simulink model "SimulinkOminidirectinalDrone"  (R2025a)
settings: Solver=VariableStepAuto  StartTime=0.0  StopTime=10.0  RelTol=1e-3
values from neighbouring files (symbols this model uses):
  Cq = 0.0013    [TiltQua.m]
  Ct = 0.013    [TiltQua.m]
  g = 9.81    [TiltQua.m]
  H = 0.05    [B_matrix.m]
  Ixx = 0.1    [TiltQua.m]
  Iyy = 0.1    [TiltQua.m]
  Izz = 0.2    [TiltQua.m]
  L = 0.25    [B_matrix.m]
  rho = 1.225    [TiltQua.m]
undefined symbols (not defined in the file or in its folder): AUM, R_rad
libraries: sharedutil x4, aerolibobsolete x1
settings Model: Creator=Nguyen_Duc  LastModifiedBy=Admin
settings RTWCC: GPUComputeCapability=3.5

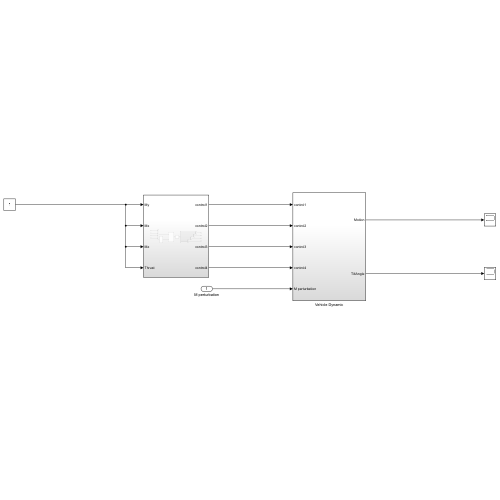
[thumbnail: Simulink's stored preview of the top-level diagram]
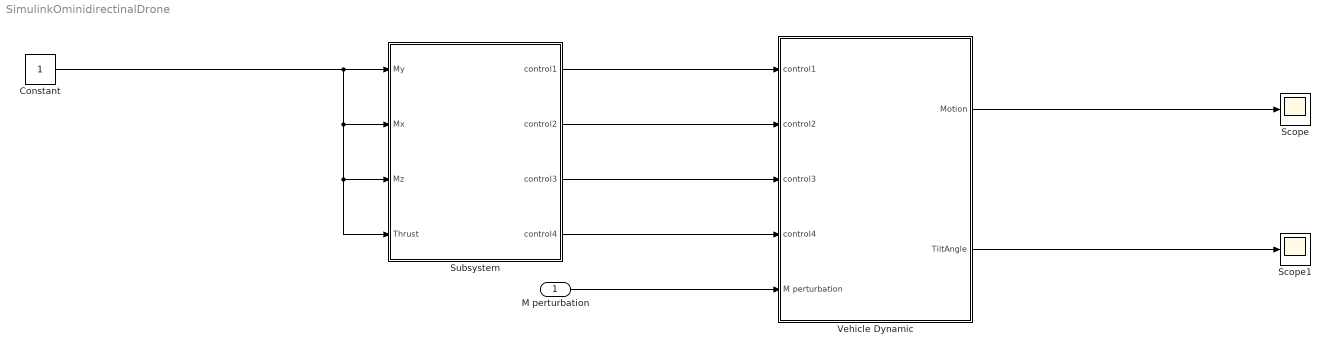
== system SimulinkOminidirectinalDrone ==
  M perturbation : Inport
  Constant : Constant
  Scope : Scope
  Scope1 : Scope
  Subsystem : Subsystem
  Vehicle Dynamic : Subsystem
  wires:
  Subsystem/1(control1) -> Vehicle Dynamic/1(control1)
  Subsystem/2(control2) -> Vehicle Dynamic/2(control2)
  Subsystem/3(control3) -> Vehicle Dynamic/3(control3)
  Subsystem/4(control4) -> Vehicle Dynamic/4(control4)
  M perturbation/1 -> Vehicle Dynamic/5(M perturbation)
  Vehicle Dynamic/1(Motion) -> Scope/1
  Vehicle Dynamic/2(TiltAngle) -> Scope1/1
  Constant/1 -> Subsystem/1(My), Subsystem/4(Thrust), Subsystem/3(Mz), Subsystem/2(Mx)

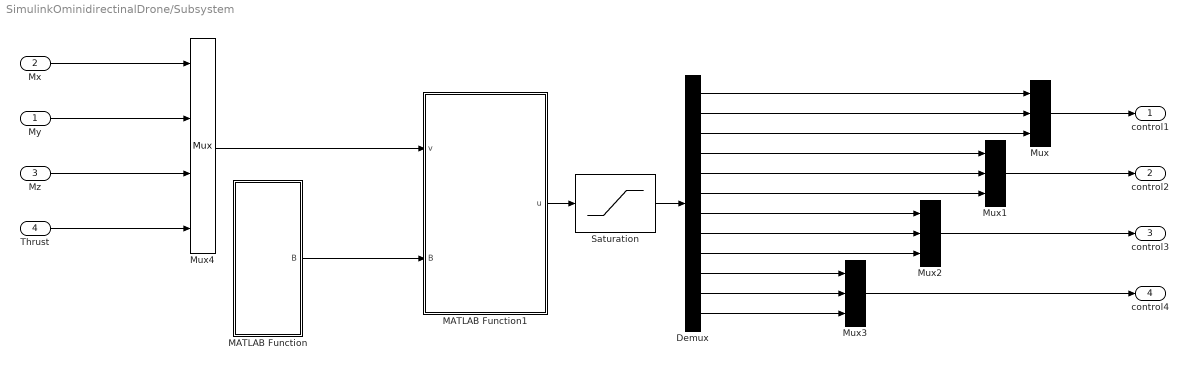
== system SimulinkOminidirectinalDrone/Subsystem ==
  My : Inport
  Mx : Inport  Port=2
  Mz : Inport  Port=3
  Thrust : Inport  Port=4
  Demux : Demux  Outputs=12
  MATLAB Function : MATLAB Function  TreatAsAtomicUnit=on
  MATLAB Function1 : MATLAB Function  TreatAsAtomicUnit=on
  Mux{,1..3} (4 alike) : Mux  Inputs=3
  Mux4 : Mux
  Saturation : Saturate  UpperLimit="[1  30*pi/180  0.2  1  30*pi/180  0.2  1  30*pi/180  0.2  1  30*pi/180  0.2]"  LowerLimit="[0 -30*pi/180 -0.2  0 -30*pi/180 -0.2  0 -30*pi/180 -0.2  0 -30*pi/180 -0.2]"
  control1 : Outport
  control2 : Outport  Port=2
  control3 : Outport  Port=3
  control4 : Outport  Port=4
  wires:
  MATLAB Function/1(B) -> MATLAB Function1/2(B)
  Mux4/1 -> MATLAB Function1/1(v)
  MATLAB Function1/1(u) -> Saturation/1
  Saturation/1 -> Demux/1
  Demux/1 -> Mux/1
  Mux/1 -> control1/1
  Demux/3 -> Mux/3
  Demux/2 -> Mux/2
  Demux/4 -> Mux1/1
  Demux/5 -> Mux1/2
  Demux/6 -> Mux1/3
  Demux/7 -> Mux2/1
  Demux/8 -> Mux2/2
  Demux/9 -> Mux2/3
  Demux/10 -> Mux3/1
  Demux/11 -> Mux3/2
  Demux/12 -> Mux3/3
  Mux1/1 -> control2/1
  Mux2/1 -> control3/1
  Mux3/1 -> control4/1
  Mx/1 -> Mux4/1
  My/1 -> Mux4/2
  Mz/1 -> Mux4/3
  Thrust/1 -> Mux4/4

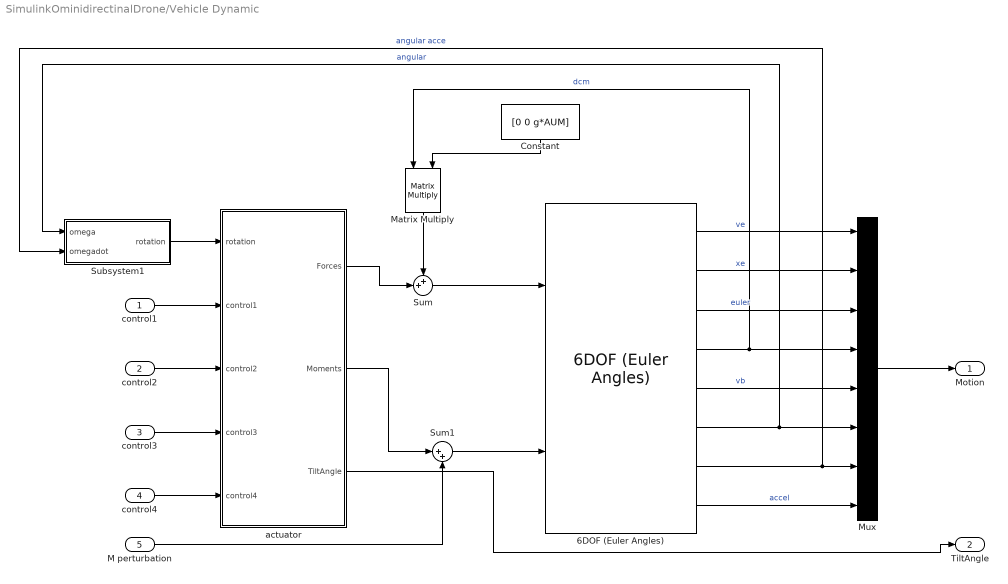
== system SimulinkOminidirectinalDrone/Vehicle Dynamic ==
  control1 : Inport
  control2 : Inport  Port=2
  control3 : Inport  Port=3
  control4 : Inport  Port=4
  M perturbation : Inport  Port=5
  6DOF (Euler Angles) : aerolibobsolete/6DOF (Euler Angles)  units=Metric (MKS)  mtype=Fixed  rep=Euler Angles  xme_0=[0 0 0]  Vm_0=[0 0 0]  eul_0=[0 0 0]  pm_0=[0 0 0]  mass_0=1.0  mass_e=0.5  mass_f=2.0  inertia=eye(3)  inertia_e=eye(3)  inertia_f=2*eye(3)  k_quat=1.0  vre_flag=on  abi_flag=off  aMode=0  xme_statename=''  Vm_statename=''  eul_statename=''  quat_statename=''  pm_statename=''  mass_statename=''
  Constant : Constant  Value=[0 0 g*AUM]
  Matrix Multiply : Product  Multiplication=Matrix(*)
  Mux : Mux  Inputs=8
  Subsystem1 : Subsystem
  Sum : Sum  Inputs=++|
  Sum1 : Sum  Inputs=|++
  actuator : Subsystem
  Motion : Outport
  TiltAngle : Outport  Port=2
  wires:
  control3/1 -> actuator/4(control3)
  M perturbation/1 -> Sum1/2
  Matrix Multiply/1 -> Sum/1
  6DOF (Euler Angles)/7 -> Subsystem1/2(omegadot), Mux/7  "angular acce"
  6DOF (Euler Angles)/3 -> Mux/3  "euler"
  Mux/1 -> Motion/1
  control1/1 -> actuator/2(control1)
  6DOF (Euler Angles)/2 -> Mux/2  "xe"
  6DOF (Euler Angles)/1 -> Mux/1  "ve"
  control2/1 -> actuator/3(control2)
  control4/1 -> actuator/5(control4)
  Constant/1 -> Matrix Multiply/2
  6DOF (Euler Angles)/8 -> Mux/8  "accel"
  6DOF (Euler Angles)/6 -> Subsystem1/1(omega), Mux/6  "angular"
  6DOF (Euler Angles)/5 -> Mux/5  "vb"
  6DOF (Euler Angles)/4 -> Matrix Multiply/1, Mux/4  "dcm"
  Sum1/1 -> 6DOF (Euler Angles)/2
  actuator/3(TiltAngle) -> TiltAngle/1
  Subsystem1/1(rotation) -> actuator/1(rotation)
  Sum/1 -> 6DOF (Euler Angles)/1
  actuator/1(Forces) -> Sum/2
  actuator/2(Moments) -> Sum1/1

== system SimulinkOminidirectinalDrone/Vehicle Dynamic/Subsystem1 ==
  omega : Inport
  omegadot : Inport  Port=2
  Demux : Demux  Outputs=3
  Demux1 : Demux  Outputs=3
  Mux1 : Mux  Inputs=6
  rotation : Outport
  wires:
  Mux1/1 -> rotation/1
  Demux/3 -> Mux1/3
  Demux1/1 -> Mux1/4
  omega/1 -> Demux/1
  Demux1/2 -> Mux1/5
  Demux/1 -> Mux1/1
  Demux/2 -> Mux1/2
  omegadot/1 -> Demux1/1
  Demux1/3 -> Mux1/6

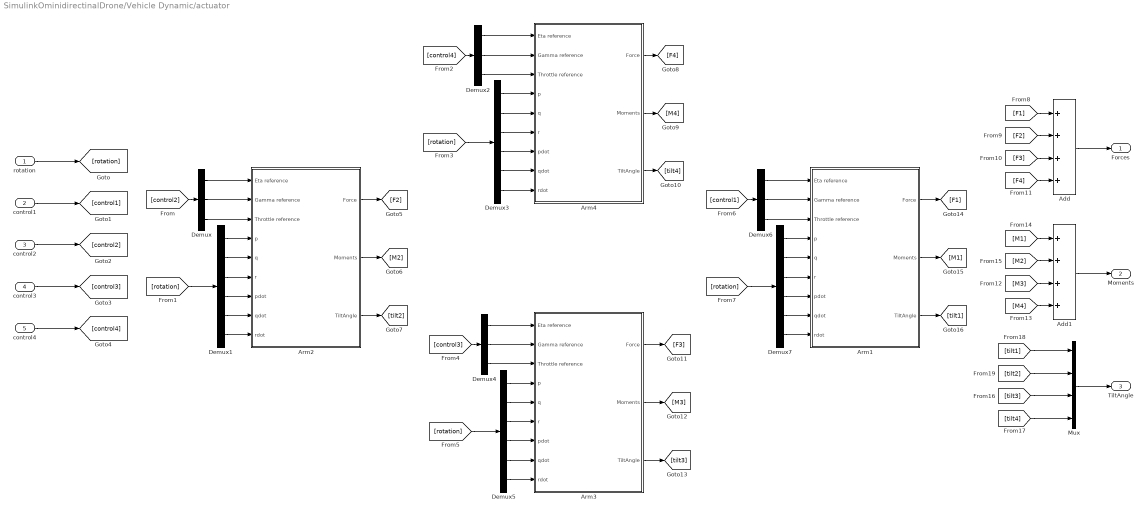
== system SimulinkOminidirectinalDrone/Vehicle Dynamic/actuator ==
  rotation : Inport
  control1 : Inport  Port=2
  control2 : Inport  Port=3
  control3 : Inport  Port=4
  control4 : Inport  Port=5
  Add : Sum  Inputs=++++
  Add1 : Sum  Inputs=++++
  Arm1 : Subsystem
  Arm2 : Subsystem
  Arm3 : Subsystem
  Arm4 : Subsystem
  Demux{,2,4,6} (4 alike) : Demux  Outputs=3
  Demux{1,3,5,7} (4 alike) : Demux  Outputs=6
  Mux : Mux
  Forces : Outport
  Moments : Outport  Port=2
  TiltAngle : Outport  Port=3
  wires:
  Demux5/3 -> Arm3/6(r)
  Demux7/6 -> Arm1/9(rdot)
  control3/1 -> [control3]
  Demux1/3 -> Arm2/6(r)
  Demux6/2 -> Arm1/2(Gamma reference)
  Add/1 -> Forces/1
  Demux4/3 -> Arm3/3(Throttle reference)
  Demux2/3 -> Arm4/3(Throttle reference)
  [F4] -> Add/4
  Arm1/3(TiltAngle) -> [tilt1]
  [tilt4] -> Mux/4
  [M3] -> Add1/3
  Demux4/2 -> Arm3/2(Gamma reference)
  Demux5/2 -> Arm3/5(q)
  [control1] -> Demux6/1
  Arm1/2(Moments) -> [M1]
  Arm3/1(Force) -> [F3]
  Demux7/3 -> Arm1/6(r)
  Demux5/5 -> Arm3/8(qdot)
  [M2] -> Add1/2
  Arm2/1(Force) -> [F2]
  Arm1/1(Force) -> [F1]
  Demux1/2 -> Arm2/5(q)
  Demux7/5 -> Arm1/8(qdot)
  Demux1/6 -> Arm2/9(rdot)
  [rotation] -> Demux3/1
  [M1] -> Add1/1
  [M4] -> Add1/4
  [control3] -> Demux4/1
  Add1/1 -> Moments/1
  Demux5/6 -> Arm3/9(rdot)
  Demux3/2 -> Arm4/5(q)
  [tilt2] -> Mux/2
  Demux1/1 -> Arm2/4(p)
  Arm4/1(Force) -> [F4]
  Demux5/4 -> Arm3/7(pdot)
  Demux3/5 -> Arm4/8(qdot)
  Demux3/4 -> Arm4/7(pdot)
  Demux3/6 -> Arm4/9(rdot)
  Demux6/1 -> Arm1/1(Eta reference)
  Demux7/2 -> Arm1/5(q)
  Arm3/2(Moments) -> [M3]
  Demux7/4 -> Arm1/7(pdot)
  Arm4/2(Moments) -> [M4]
  control1/1 -> [control1]
  Demux2/2 -> Arm4/2(Gamma reference)
  Arm2/3(TiltAngle) -> [tilt2]
  [control4] -> Demux2/1
  Demux3/3 -> Arm4/6(r)
  Demux3/1 -> Arm4/4(p)
  Demux6/3 -> Arm1/3(Throttle reference)
  Arm4/3(TiltAngle) -> [tilt4]
  Demux2/1 -> Arm4/1(Eta reference)
  Demux5/1 -> Arm3/4(p)
  Demux/2 -> Arm2/2(Gamma reference)
  [control2] -> Demux/1
  control2/1 -> [control2]
  Demux7/1 -> Arm1/4(p)
  Arm2/2(Moments) -> [M2]
  [rotation] -> Demux1/1
  Arm3/3(TiltAngle) -> [tilt3]
  [rotation] -> Demux7/1
  Demux/1 -> Arm2/1(Eta reference)
  Demux4/1 -> Arm3/1(Eta reference)
  [rotation] -> Demux5/1
  Demux1/4 -> Arm2/7(pdot)
  rotation/1 -> [rotation]
  Demux/3 -> Arm2/3(Throttle reference)
  control4/1 -> [control4]
  Demux1/5 -> Arm2/8(qdot)
  Mux/1 -> TiltAngle/1
  [F3] -> Add/3
  [F1] -> Add/1
  [tilt1] -> Mux/1
  [tilt3] -> Mux/3
  [F2] -> Add/2

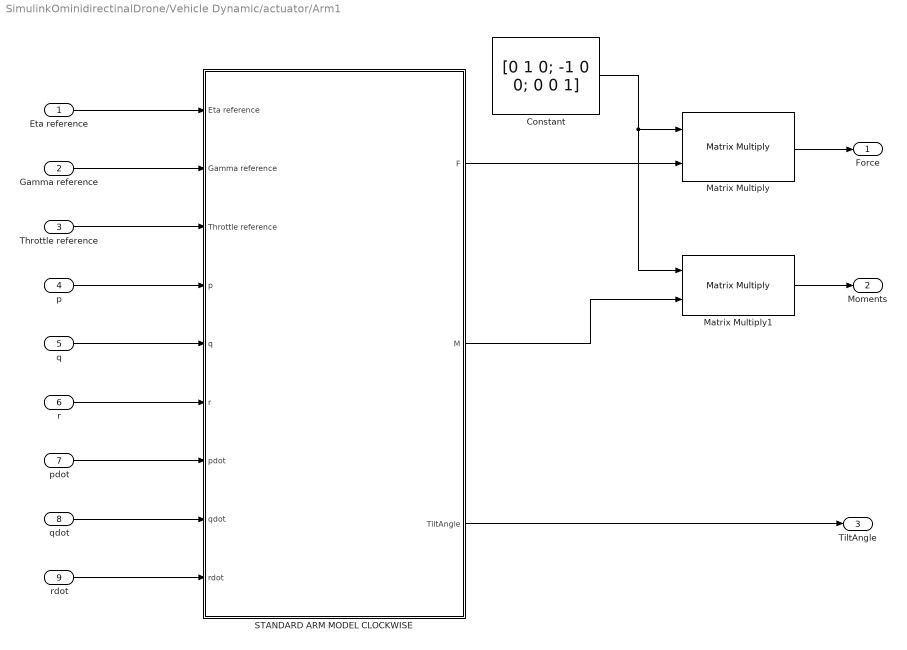
== system SimulinkOminidirectinalDrone/Vehicle Dynamic/actuator/Arm1 ==
  Eta reference : Inport
  Gamma reference : Inport  Port=2
  Throttle reference : Inport  Port=3
  p : Inport  Port=4
  q : Inport  Port=5
  r : Inport  Port=6
  pdot : Inport  Port=7
  qdot : Inport  Port=8
  rdot : Inport  Port=9
  Constant : Constant  Value=[0 1 0; -1 0 0; 0 0 1]
  Matrix Multiply : Product  Multiplication=Matrix(*)
  Matrix Multiply1 : Product  Multiplication=Matrix(*)
  STANDARD ARM MODEL CLOCKWISE : Subsystem
  Force : Outport
  Moments : Outport  Port=2
  TiltAngle : Outport  Port=3
  wires:
  Gamma reference/1 -> STANDARD ARM MODEL CLOCKWISE/2(Gamma reference)
  Eta reference/1 -> STANDARD ARM MODEL CLOCKWISE/1(Eta reference)
  Matrix Multiply1/1 -> Moments/1
  STANDARD ARM MODEL CLOCKWISE/1(F) -> Matrix Multiply/2
  Throttle reference/1 -> STANDARD ARM MODEL CLOCKWISE/3(Throttle reference)
  r/1 -> STANDARD ARM MODEL CLOCKWISE/6(r)
  p/1 -> STANDARD ARM MODEL CLOCKWISE/4(p)
  q/1 -> STANDARD ARM MODEL CLOCKWISE/5(q)
  STANDARD ARM MODEL CLOCKWISE/2(M) -> Matrix Multiply1/2
  pdot/1 -> STANDARD ARM MODEL CLOCKWISE/7(pdot)
  qdot/1 -> STANDARD ARM MODEL CLOCKWISE/8(qdot)
  rdot/1 -> STANDARD ARM MODEL CLOCKWISE/9(rdot)
  Constant/1 -> Matrix Multiply1/1, Matrix Multiply/1
  Matrix Multiply/1 -> Force/1
  STANDARD ARM MODEL CLOCKWISE/3(TiltAngle) -> TiltAngle/1

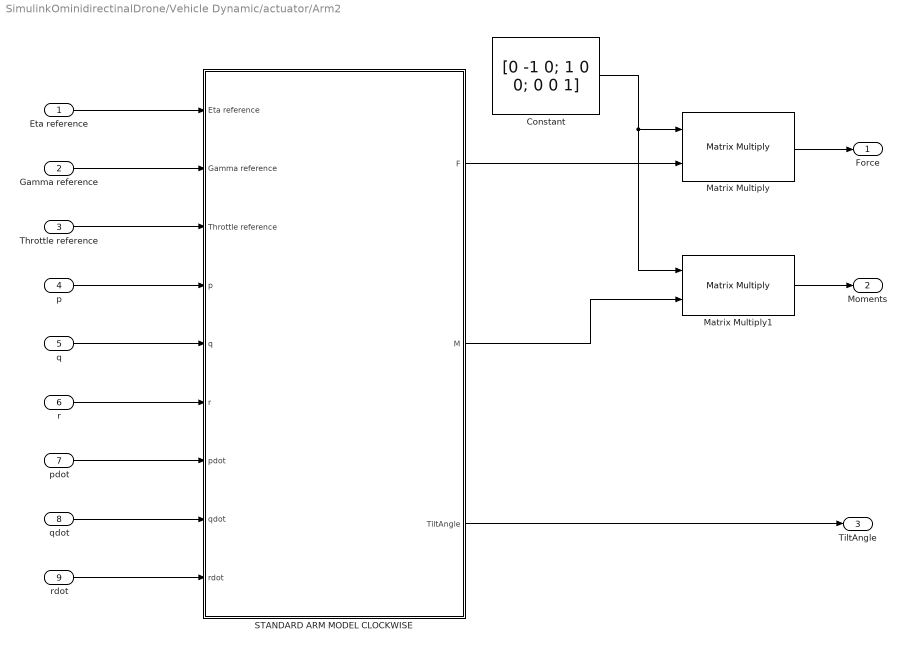
== system SimulinkOminidirectinalDrone/Vehicle Dynamic/actuator/Arm2 ==
  Eta reference : Inport
  Gamma reference : Inport  Port=2
  Throttle reference : Inport  Port=3
  p : Inport  Port=4
  q : Inport  Port=5
  r : Inport  Port=6
  pdot : Inport  Port=7
  qdot : Inport  Port=8
  rdot : Inport  Port=9
  Constant : Constant  Value=[0 -1 0; 1 0 0; 0 0 1]
  Matrix Multiply : Product  Multiplication=Matrix(*)
  Matrix Multiply1 : Product  Multiplication=Matrix(*)
  STANDARD ARM MODEL CLOCKWISE : Subsystem
  Force : Outport
  Moments : Outport  Port=2
  TiltAngle : Outport  Port=3
  wires:
  Gamma reference/1 -> STANDARD ARM MODEL CLOCKWISE/2(Gamma reference)
  Eta reference/1 -> STANDARD ARM MODEL CLOCKWISE/1(Eta reference)
  Matrix Multiply1/1 -> Moments/1
  STANDARD ARM MODEL CLOCKWISE/1(F) -> Matrix Multiply/2
  Throttle reference/1 -> STANDARD ARM MODEL CLOCKWISE/3(Throttle reference)
  r/1 -> STANDARD ARM MODEL CLOCKWISE/6(r)
  p/1 -> STANDARD ARM MODEL CLOCKWISE/4(p)
  q/1 -> STANDARD ARM MODEL CLOCKWISE/5(q)
  STANDARD ARM MODEL CLOCKWISE/2(M) -> Matrix Multiply1/2
  pdot/1 -> STANDARD ARM MODEL CLOCKWISE/7(pdot)
  qdot/1 -> STANDARD ARM MODEL CLOCKWISE/8(qdot)
  rdot/1 -> STANDARD ARM MODEL CLOCKWISE/9(rdot)
  Constant/1 -> Matrix Multiply1/1, Matrix Multiply/1
  Matrix Multiply/1 -> Force/1
  STANDARD ARM MODEL CLOCKWISE/3(TiltAngle) -> TiltAngle/1

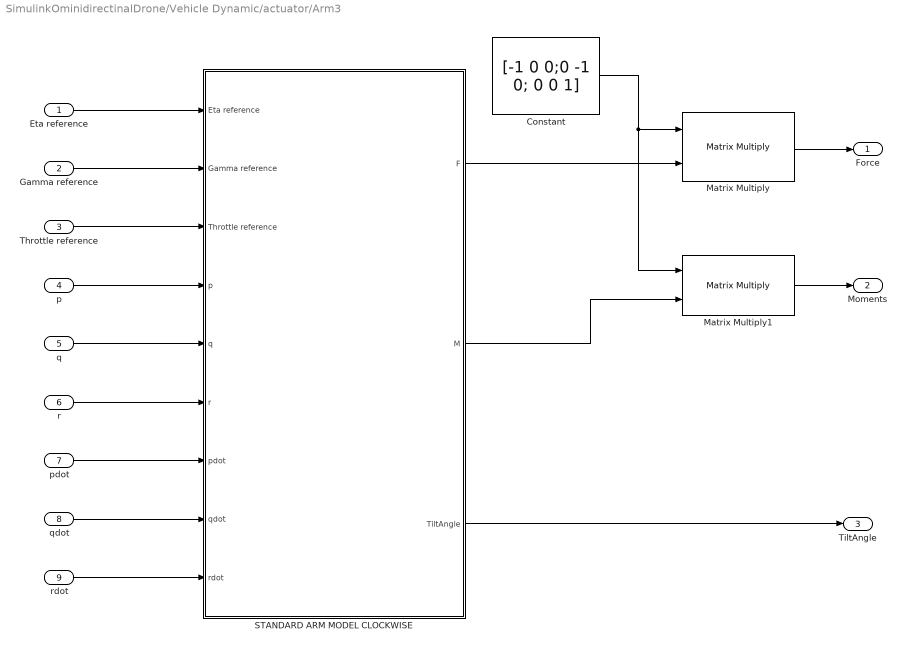
== system SimulinkOminidirectinalDrone/Vehicle Dynamic/actuator/Arm3 ==
  Eta reference : Inport
  Gamma reference : Inport  Port=2
  Throttle reference : Inport  Port=3
  p : Inport  Port=4
  q : Inport  Port=5
  r : Inport  Port=6
  pdot : Inport  Port=7
  qdot : Inport  Port=8
  rdot : Inport  Port=9
  Constant : Constant  Value=[-1 0 0;0 -1 0; 0 0 1]
  Matrix Multiply : Product  Multiplication=Matrix(*)
  Matrix Multiply1 : Product  Multiplication=Matrix(*)
  STANDARD ARM MODEL CLOCKWISE : Subsystem
  Force : Outport
  Moments : Outport  Port=2
  TiltAngle : Outport  Port=3
  wires:
  Gamma reference/1 -> STANDARD ARM MODEL CLOCKWISE/2(Gamma reference)
  Eta reference/1 -> STANDARD ARM MODEL CLOCKWISE/1(Eta reference)
  Matrix Multiply1/1 -> Moments/1
  STANDARD ARM MODEL CLOCKWISE/1(F) -> Matrix Multiply/2
  Throttle reference/1 -> STANDARD ARM MODEL CLOCKWISE/3(Throttle reference)
  r/1 -> STANDARD ARM MODEL CLOCKWISE/6(r)
  p/1 -> STANDARD ARM MODEL CLOCKWISE/4(p)
  q/1 -> STANDARD ARM MODEL CLOCKWISE/5(q)
  STANDARD ARM MODEL CLOCKWISE/2(M) -> Matrix Multiply1/2
  pdot/1 -> STANDARD ARM MODEL CLOCKWISE/7(pdot)
  qdot/1 -> STANDARD ARM MODEL CLOCKWISE/8(qdot)
  rdot/1 -> STANDARD ARM MODEL CLOCKWISE/9(rdot)
  Constant/1 -> Matrix Multiply1/1, Matrix Multiply/1
  Matrix Multiply/1 -> Force/1
  STANDARD ARM MODEL CLOCKWISE/3(TiltAngle) -> TiltAngle/1

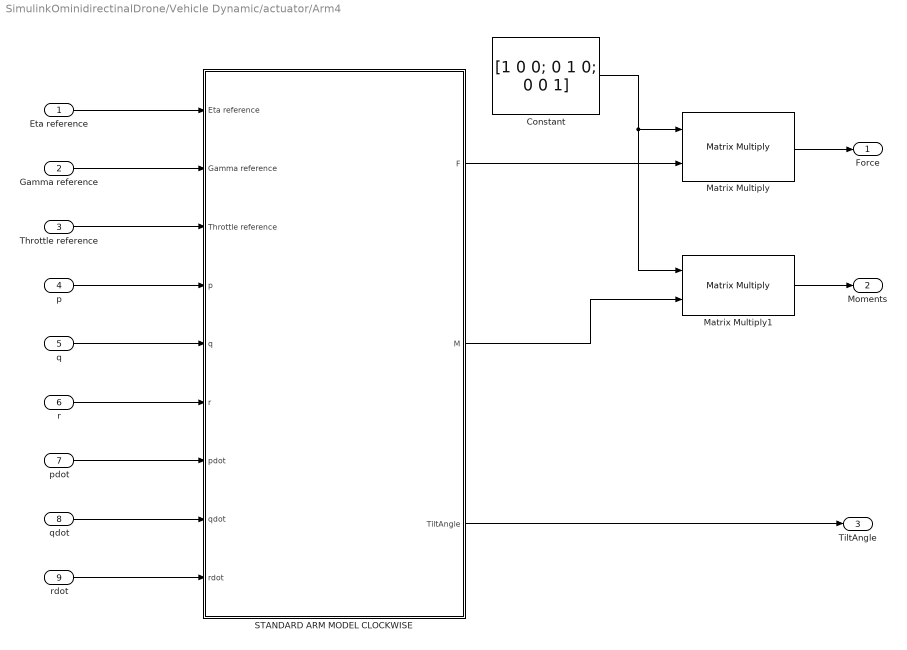
== system SimulinkOminidirectinalDrone/Vehicle Dynamic/actuator/Arm4 ==
  Eta reference : Inport
  Gamma reference : Inport  Port=2
  Throttle reference : Inport  Port=3
  p : Inport  Port=4
  q : Inport  Port=5
  r : Inport  Port=6
  pdot : Inport  Port=7
  qdot : Inport  Port=8
  rdot : Inport  Port=9
  Constant : Constant  Value=[1 0 0; 0 1 0; 0 0 1]
  Matrix Multiply : Product  Multiplication=Matrix(*)
  Matrix Multiply1 : Product  Multiplication=Matrix(*)
  STANDARD ARM MODEL CLOCKWISE : Subsystem
  Force : Outport
  Moments : Outport  Port=2
  TiltAngle : Outport  Port=3
  wires:
  Gamma reference/1 -> STANDARD ARM MODEL CLOCKWISE/2(Gamma reference)
  Eta reference/1 -> STANDARD ARM MODEL CLOCKWISE/1(Eta reference)
  Matrix Multiply1/1 -> Moments/1
  STANDARD ARM MODEL CLOCKWISE/1(F) -> Matrix Multiply/2
  Throttle reference/1 -> STANDARD ARM MODEL CLOCKWISE/3(Throttle reference)
  r/1 -> STANDARD ARM MODEL CLOCKWISE/6(r)
  p/1 -> STANDARD ARM MODEL CLOCKWISE/4(p)
  q/1 -> STANDARD ARM MODEL CLOCKWISE/5(q)
  STANDARD ARM MODEL CLOCKWISE/2(M) -> Matrix Multiply1/2
  pdot/1 -> STANDARD ARM MODEL CLOCKWISE/7(pdot)
  qdot/1 -> STANDARD ARM MODEL CLOCKWISE/8(qdot)
  rdot/1 -> STANDARD ARM MODEL CLOCKWISE/9(rdot)
  Constant/1 -> Matrix Multiply1/1, Matrix Multiply/1
  Matrix Multiply/1 -> Force/1
  STANDARD ARM MODEL CLOCKWISE/3(TiltAngle) -> TiltAngle/1

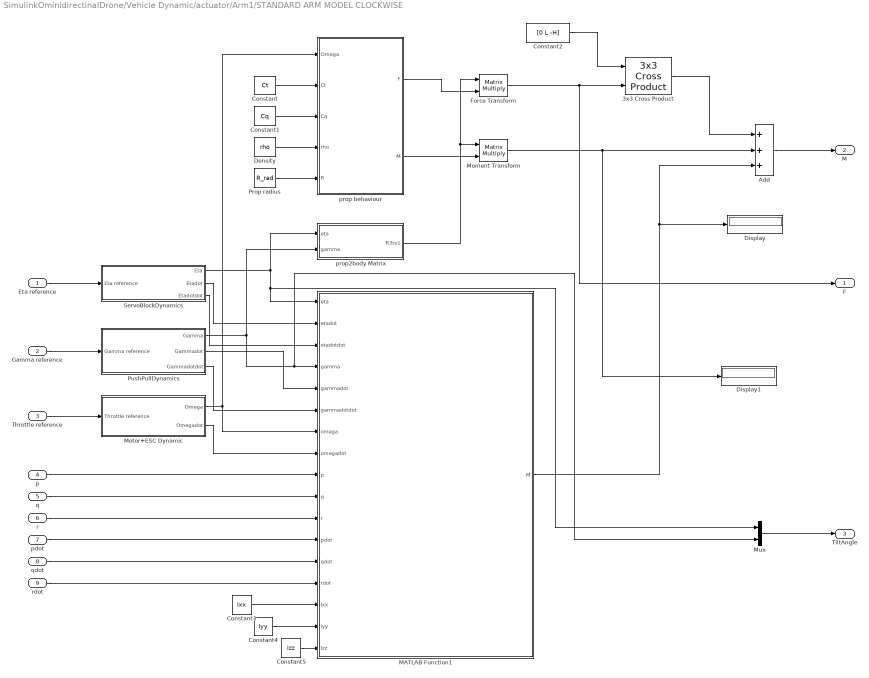
== system SimulinkOminidirectinalDrone/Vehicle Dynamic/actuator/Arm1/STANDARD ARM MODEL CLOCKWISE ==
  Eta reference : Inport
  Gamma reference : Inport  Port=2
  Throttle reference : Inport  Port=3
  p : Inport  Port=4
  q : Inport  Port=5
  r : Inport  Port=6
  pdot : Inport  Port=7
  qdot : Inport  Port=8
  rdot : Inport  Port=9
  3x3 Cross Product : sharedutil/3x3 Cross Product  aMode=aMode
      settings: LibrarySourceBlock=aerolibutil/3x3 Cross Product
  Add : Sum  Inputs=+++
  Constant : Constant  Value=Ct
  Constant1 : Constant  Value=Cq
  Constant2 : Constant  Value=[0 L -H]
  Constant3 : Constant  Value=Ixx
  Constant4 : Constant  Value=Iyy
  Constant5 : Constant  Value=Izz
  Density : Constant  Value=rho
  Display : Display
  Display1 : Display
  Force Transform : Product  Multiplication=Matrix(*)
  MATLAB Function1 : MATLAB Function  TreatAsAtomicUnit=on
  Moment Transform : Product  Multiplication=Matrix(*)
  Motor+ESC Dynamic : Subsystem
  Mux : Mux  Inputs=2
  Prop radius : Constant  Value=R_rad
  PushPullDynamics : Subsystem
  ServoBlockDynamics : Subsystem
  prop behaviour : MATLAB Function  TreatAsAtomicUnit=on
  prop2body Matrix : MATLAB Function  TreatAsAtomicUnit=on
  F : Outport
  M : Outport  Port=2
  TiltAngle : Outport  Port=3
  wires:
  Motor+ESC Dynamic/2(Omegadot) -> MATLAB Function1/8(omegadot)
  PushPullDynamics/3(Gammadotdot) -> MATLAB Function1/6(gammadotdot)
  Constant5/1 -> MATLAB Function1/17(Izz)
  Constant4/1 -> MATLAB Function1/16(Iyy)
  p/1 -> MATLAB Function1/9(p)
  prop2body Matrix/1(R3to1) -> Moment Transform/1, Force Transform/1
  Moment Transform/1 -> Display1/1, Add/2
  Prop radius/1 -> prop behaviour/5(R)
  Gamma reference/1 -> PushPullDynamics/1(Gamma reference)
  qdot/1 -> MATLAB Function1/13(qdot)
  Constant1/1 -> prop behaviour/3(Cq)
  Throttle reference/1 -> Motor+ESC Dynamic/1(Throttle reference)
  3x3 Cross Product/1 -> Add/1
  q/1 -> MATLAB Function1/10(q)
  Density/1 -> prop behaviour/4(rho)
  Motor+ESC Dynamic/1(Omega) -> MATLAB Function1/7(omega), prop behaviour/1(Omega)
  ServoBlockDynamics/3(Etadotdot) -> MATLAB Function1/3(etadotdot)
  prop behaviour/2(M) -> Moment Transform/2
  Constant3/1 -> MATLAB Function1/15(Ixx)
  PushPullDynamics/1(Gamma) -> Mux/2, MATLAB Function1/4(gamma), prop2body Matrix/2(gamma)
  Constant2/1 -> 3x3 Cross Product/1
  Force Transform/1 -> F/1, 3x3 Cross Product/2
  MATLAB Function1/1(M) -> Display/1, Add/3
  ServoBlockDynamics/1(Eta) -> Mux/1, MATLAB Function1/1(eta), prop2body Matrix/1(eta)
  r/1 -> MATLAB Function1/11(r)
  rdot/1 -> MATLAB Function1/14(rdot)
  Eta reference/1 -> ServoBlockDynamics/1(Eta reference)
  Mux/1 -> TiltAngle/1
  PushPullDynamics/2(Gammadot) -> MATLAB Function1/5(gammadot)
  pdot/1 -> MATLAB Function1/12(pdot)
  prop behaviour/1(F) -> Force Transform/2
  Constant/1 -> prop behaviour/2(Ct)
  Add/1 -> M/1
  ServoBlockDynamics/2(Etadot) -> MATLAB Function1/2(etadot)

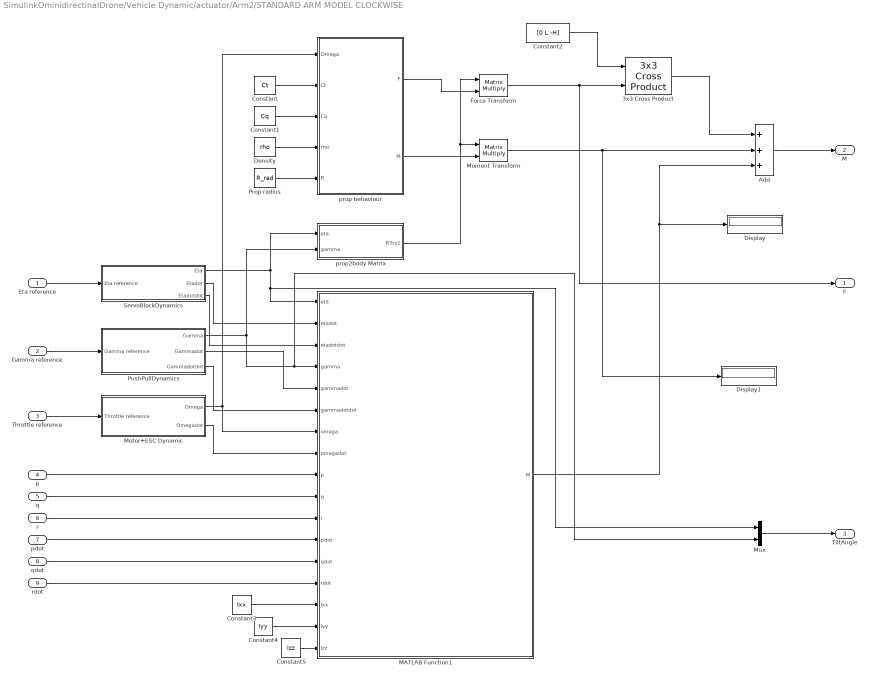
== system SimulinkOminidirectinalDrone/Vehicle Dynamic/actuator/Arm2/STANDARD ARM MODEL CLOCKWISE ==
  Eta reference : Inport
  Gamma reference : Inport  Port=2
  Throttle reference : Inport  Port=3
  p : Inport  Port=4
  q : Inport  Port=5
  r : Inport  Port=6
  pdot : Inport  Port=7
  qdot : Inport  Port=8
  rdot : Inport  Port=9
  3x3 Cross Product : sharedutil/3x3 Cross Product  aMode=aMode
      settings: LibrarySourceBlock=aerolibutil/3x3 Cross Product
  Add : Sum  Inputs=+++
  Constant : Constant  Value=Ct
  Constant1 : Constant  Value=Cq
  Constant2 : Constant  Value=[0 L -H]
  Constant3 : Constant  Value=Ixx
  Constant4 : Constant  Value=Iyy
  Constant5 : Constant  Value=Izz
  Density : Constant  Value=rho
  Display : Display
  Display1 : Display
  Force Transform : Product  Multiplication=Matrix(*)
  MATLAB Function1 : MATLAB Function  TreatAsAtomicUnit=on
  Moment Transform : Product  Multiplication=Matrix(*)
  Motor+ESC Dynamic : Subsystem
  Mux : Mux  Inputs=2
  Prop radius : Constant  Value=R_rad
  PushPullDynamics : Subsystem
  ServoBlockDynamics : Subsystem
  prop behaviour : MATLAB Function  TreatAsAtomicUnit=on
  prop2body Matrix : MATLAB Function  TreatAsAtomicUnit=on
  F : Outport
  M : Outport  Port=2
  TiltAngle : Outport  Port=3
  wires:
  Motor+ESC Dynamic/2(Omegadot) -> MATLAB Function1/8(omegadot)
  PushPullDynamics/3(Gammadotdot) -> MATLAB Function1/6(gammadotdot)
  Constant5/1 -> MATLAB Function1/17(Izz)
  Constant4/1 -> MATLAB Function1/16(Iyy)
  p/1 -> MATLAB Function1/9(p)
  prop2body Matrix/1(R3to1) -> Moment Transform/1, Force Transform/1
  Moment Transform/1 -> Display1/1, Add/2
  Prop radius/1 -> prop behaviour/5(R)
  Gamma reference/1 -> PushPullDynamics/1(Gamma reference)
  qdot/1 -> MATLAB Function1/13(qdot)
  Constant1/1 -> prop behaviour/3(Cq)
  Throttle reference/1 -> Motor+ESC Dynamic/1(Throttle reference)
  3x3 Cross Product/1 -> Add/1
  q/1 -> MATLAB Function1/10(q)
  Density/1 -> prop behaviour/4(rho)
  Motor+ESC Dynamic/1(Omega) -> MATLAB Function1/7(omega), prop behaviour/1(Omega)
  ServoBlockDynamics/3(Etadotdot) -> MATLAB Function1/3(etadotdot)
  prop behaviour/2(M) -> Moment Transform/2
  Constant3/1 -> MATLAB Function1/15(Ixx)
  PushPullDynamics/1(Gamma) -> Mux/2, MATLAB Function1/4(gamma), prop2body Matrix/2(gamma)
  Constant2/1 -> 3x3 Cross Product/1
  Force Transform/1 -> F/1, 3x3 Cross Product/2
  MATLAB Function1/1(M) -> Display/1, Add/3
  ServoBlockDynamics/1(Eta) -> Mux/1, MATLAB Function1/1(eta), prop2body Matrix/1(eta)
  r/1 -> MATLAB Function1/11(r)
  rdot/1 -> MATLAB Function1/14(rdot)
  Eta reference/1 -> ServoBlockDynamics/1(Eta reference)
  Mux/1 -> TiltAngle/1
  PushPullDynamics/2(Gammadot) -> MATLAB Function1/5(gammadot)
  pdot/1 -> MATLAB Function1/12(pdot)
  prop behaviour/1(F) -> Force Transform/2
  Constant/1 -> prop behaviour/2(Ct)
  Add/1 -> M/1
  ServoBlockDynamics/2(Etadot) -> MATLAB Function1/2(etadot)

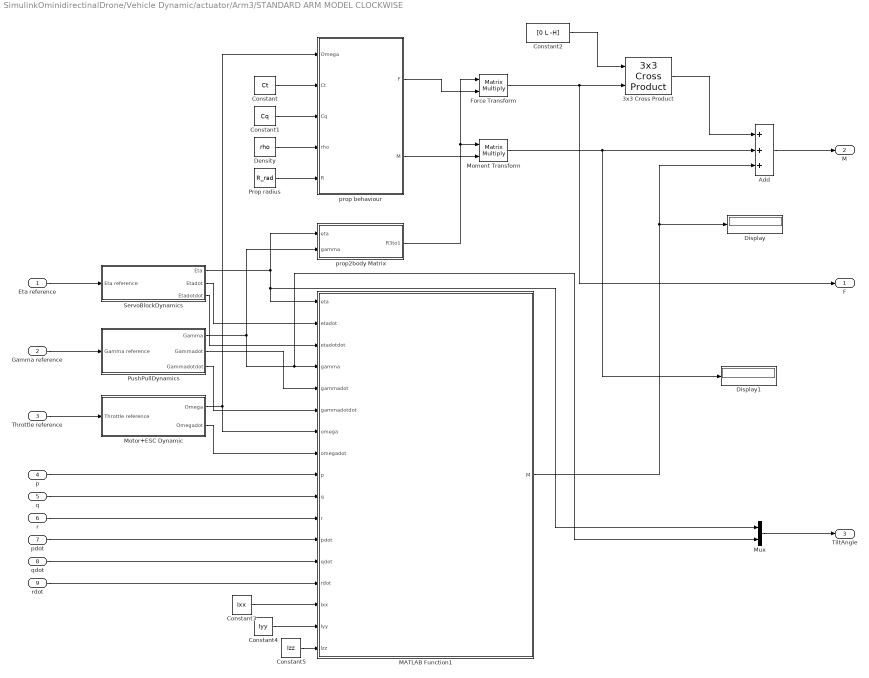
== system SimulinkOminidirectinalDrone/Vehicle Dynamic/actuator/Arm3/STANDARD ARM MODEL CLOCKWISE ==
  Eta reference : Inport
  Gamma reference : Inport  Port=2
  Throttle reference : Inport  Port=3
  p : Inport  Port=4
  q : Inport  Port=5
  r : Inport  Port=6
  pdot : Inport  Port=7
  qdot : Inport  Port=8
  rdot : Inport  Port=9
  3x3 Cross Product : sharedutil/3x3 Cross Product  aMode=aMode
      settings: LibrarySourceBlock=aerolibutil/3x3 Cross Product
  Add : Sum  Inputs=+++
  Constant : Constant  Value=Ct
  Constant1 : Constant  Value=Cq
  Constant2 : Constant  Value=[0 L -H]
  Constant3 : Constant  Value=Ixx
  Constant4 : Constant  Value=Iyy
  Constant5 : Constant  Value=Izz
  Density : Constant  Value=rho
  Display : Display
  Display1 : Display
  Force Transform : Product  Multiplication=Matrix(*)
  MATLAB Function1 : MATLAB Function  TreatAsAtomicUnit=on
  Moment Transform : Product  Multiplication=Matrix(*)
  Motor+ESC Dynamic : Subsystem
  Mux : Mux  Inputs=2
  Prop radius : Constant  Value=R_rad
  PushPullDynamics : Subsystem
  ServoBlockDynamics : Subsystem
  prop behaviour : MATLAB Function  TreatAsAtomicUnit=on
  prop2body Matrix : MATLAB Function  TreatAsAtomicUnit=on
  F : Outport
  M : Outport  Port=2
  TiltAngle : Outport  Port=3
  wires:
  Motor+ESC Dynamic/2(Omegadot) -> MATLAB Function1/8(omegadot)
  PushPullDynamics/3(Gammadotdot) -> MATLAB Function1/6(gammadotdot)
  Constant5/1 -> MATLAB Function1/17(Izz)
  Constant4/1 -> MATLAB Function1/16(Iyy)
  p/1 -> MATLAB Function1/9(p)
  prop2body Matrix/1(R3to1) -> Moment Transform/1, Force Transform/1
  Moment Transform/1 -> Display1/1, Add/2
  Prop radius/1 -> prop behaviour/5(R)
  Gamma reference/1 -> PushPullDynamics/1(Gamma reference)
  qdot/1 -> MATLAB Function1/13(qdot)
  Constant1/1 -> prop behaviour/3(Cq)
  Throttle reference/1 -> Motor+ESC Dynamic/1(Throttle reference)
  3x3 Cross Product/1 -> Add/1
  q/1 -> MATLAB Function1/10(q)
  Density/1 -> prop behaviour/4(rho)
  Motor+ESC Dynamic/1(Omega) -> MATLAB Function1/7(omega), prop behaviour/1(Omega)
  ServoBlockDynamics/3(Etadotdot) -> MATLAB Function1/3(etadotdot)
  prop behaviour/2(M) -> Moment Transform/2
  Constant3/1 -> MATLAB Function1/15(Ixx)
  PushPullDynamics/1(Gamma) -> Mux/2, MATLAB Function1/4(gamma), prop2body Matrix/2(gamma)
  Constant2/1 -> 3x3 Cross Product/1
  Force Transform/1 -> F/1, 3x3 Cross Product/2
  MATLAB Function1/1(M) -> Display/1, Add/3
  ServoBlockDynamics/1(Eta) -> Mux/1, MATLAB Function1/1(eta), prop2body Matrix/1(eta)
  r/1 -> MATLAB Function1/11(r)
  rdot/1 -> MATLAB Function1/14(rdot)
  Eta reference/1 -> ServoBlockDynamics/1(Eta reference)
  Mux/1 -> TiltAngle/1
  PushPullDynamics/2(Gammadot) -> MATLAB Function1/5(gammadot)
  pdot/1 -> MATLAB Function1/12(pdot)
  prop behaviour/1(F) -> Force Transform/2
  Constant/1 -> prop behaviour/2(Ct)
  Add/1 -> M/1
  ServoBlockDynamics/2(Etadot) -> MATLAB Function1/2(etadot)

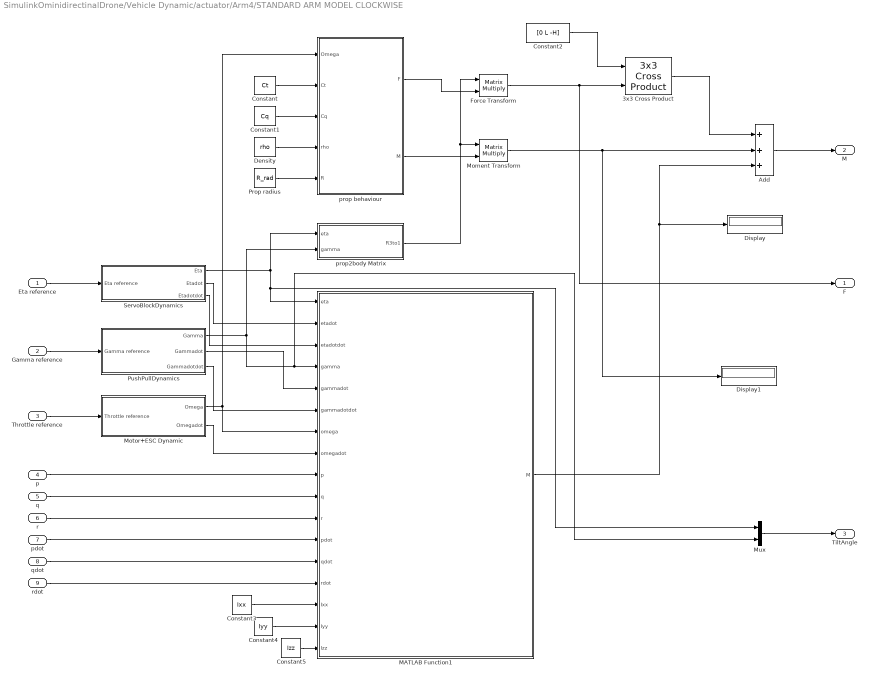
== system SimulinkOminidirectinalDrone/Vehicle Dynamic/actuator/Arm4/STANDARD ARM MODEL CLOCKWISE ==
  Eta reference : Inport
  Gamma reference : Inport  Port=2
  Throttle reference : Inport  Port=3
  p : Inport  Port=4
  q : Inport  Port=5
  r : Inport  Port=6
  pdot : Inport  Port=7
  qdot : Inport  Port=8
  rdot : Inport  Port=9
  3x3 Cross Product : sharedutil/3x3 Cross Product  aMode=aMode
      settings: LibrarySourceBlock=aerolibutil/3x3 Cross Product
  Add : Sum  Inputs=+++
  Constant : Constant  Value=Ct
  Constant1 : Constant  Value=Cq
  Constant2 : Constant  Value=[0 L -H]
  Constant3 : Constant  Value=Ixx
  Constant4 : Constant  Value=Iyy
  Constant5 : Constant  Value=Izz
  Density : Constant  Value=rho
  Display : Display
  Display1 : Display
  Force Transform : Product  Multiplication=Matrix(*)
  MATLAB Function1 : MATLAB Function  TreatAsAtomicUnit=on
  Moment Transform : Product  Multiplication=Matrix(*)
  Motor+ESC Dynamic : Subsystem
  Mux : Mux  Inputs=2
  Prop radius : Constant  Value=R_rad
  PushPullDynamics : Subsystem
  ServoBlockDynamics : Subsystem
  prop behaviour : MATLAB Function  TreatAsAtomicUnit=on
  prop2body Matrix : MATLAB Function  TreatAsAtomicUnit=on
  F : Outport
  M : Outport  Port=2
  TiltAngle : Outport  Port=3
  wires:
  Motor+ESC Dynamic/2(Omegadot) -> MATLAB Function1/8(omegadot)
  PushPullDynamics/3(Gammadotdot) -> MATLAB Function1/6(gammadotdot)
  Constant5/1 -> MATLAB Function1/17(Izz)
  Constant4/1 -> MATLAB Function1/16(Iyy)
  p/1 -> MATLAB Function1/9(p)
  prop2body Matrix/1(R3to1) -> Moment Transform/1, Force Transform/1
  Moment Transform/1 -> Display1/1, Add/2
  Prop radius/1 -> prop behaviour/5(R)
  Gamma reference/1 -> PushPullDynamics/1(Gamma reference)
  qdot/1 -> MATLAB Function1/13(qdot)
  Constant1/1 -> prop behaviour/3(Cq)
  Throttle reference/1 -> Motor+ESC Dynamic/1(Throttle reference)
  3x3 Cross Product/1 -> Add/1
  q/1 -> MATLAB Function1/10(q)
  Density/1 -> prop behaviour/4(rho)
  Motor+ESC Dynamic/1(Omega) -> MATLAB Function1/7(omega), prop behaviour/1(Omega)
  ServoBlockDynamics/3(Etadotdot) -> MATLAB Function1/3(etadotdot)
  prop behaviour/2(M) -> Moment Transform/2
  Constant3/1 -> MATLAB Function1/15(Ixx)
  PushPullDynamics/1(Gamma) -> Mux/2, MATLAB Function1/4(gamma), prop2body Matrix/2(gamma)
  Constant2/1 -> 3x3 Cross Product/1
  Force Transform/1 -> F/1, 3x3 Cross Product/2
  MATLAB Function1/1(M) -> Display/1, Add/3
  ServoBlockDynamics/1(Eta) -> Mux/1, MATLAB Function1/1(eta), prop2body Matrix/1(eta)
  r/1 -> MATLAB Function1/11(r)
  rdot/1 -> MATLAB Function1/14(rdot)
  Eta reference/1 -> ServoBlockDynamics/1(Eta reference)
  Mux/1 -> TiltAngle/1
  PushPullDynamics/2(Gammadot) -> MATLAB Function1/5(gammadot)
  pdot/1 -> MATLAB Function1/12(pdot)
  prop behaviour/1(F) -> Force Transform/2
  Constant/1 -> prop behaviour/2(Ct)
  Add/1 -> M/1
  ServoBlockDynamics/2(Etadot) -> MATLAB Function1/2(etadot)

== system SimulinkOminidirectinalDrone/Vehicle Dynamic/actuator/Arm1/STANDARD ARM MODEL CLOCKWISE/Motor+ESC Dynamic ==
  Throttle reference : Inport
  Derivative : Derivative
  G Motor : TransferFcn  Numerator=[9.19]  Denominator=[0.16 1]
  Transport Delay : TransportDelay  DelayTime=0.035
  Omega : Outport
  Omegadot : Outport  Port=2
  wires:
  Transport Delay/1 -> Omega/1, Derivative/1
  Throttle reference/1 -> G Motor/1
  G Motor/1 -> Transport Delay/1
  Derivative/1 -> Omegadot/1

== system SimulinkOminidirectinalDrone/Vehicle Dynamic/actuator/Arm1/STANDARD ARM MODEL CLOCKWISE/PushPullDynamics ==
  Gamma reference : Inport
  Derivative : Derivative
  Derivative1 : Derivative
  G pushpull : TransferFcn  Numerator=[1212.73]  Denominator=[1 51.105 1212.73]
  Gamma : Outport
  Gammadot : Outport  Port=2
  Gammadotdot : Outport  Port=3
  wires:
  Derivative/1 -> Gammadot/1, Derivative1/1
  Derivative1/1 -> Gammadotdot/1
  Gamma reference/1 -> G pushpull/1
  G pushpull/1 -> Gamma/1, Derivative/1

== system SimulinkOminidirectinalDrone/Vehicle Dynamic/actuator/Arm1/STANDARD ARM MODEL CLOCKWISE/ServoBlockDynamics ==
  Eta reference : Inport
  Derivative : Derivative
  Derivative1 : Derivative
  G Servoblock : TransferFcn  Numerator=[1228.05]  Denominator=[1 49.1806 1228.05]
  Eta : Outport
  Etadot : Outport  Port=2
  Etadotdot : Outport  Port=3
  wires:
  Derivative/1 -> Etadot/1, Derivative1/1
  Derivative1/1 -> Etadotdot/1
  Eta reference/1 -> G Servoblock/1
  G Servoblock/1 -> Eta/1, Derivative/1

== system SimulinkOminidirectinalDrone/Vehicle Dynamic/actuator/Arm2/STANDARD ARM MODEL CLOCKWISE/Motor+ESC Dynamic ==
  Throttle reference : Inport
  Derivative : Derivative
  G Motor : TransferFcn  Numerator=[9.19]  Denominator=[0.16 1]
  Transport Delay : TransportDelay  DelayTime=0.035
  Omega : Outport
  Omegadot : Outport  Port=2
  wires:
  Transport Delay/1 -> Omega/1, Derivative/1
  Throttle reference/1 -> G Motor/1
  G Motor/1 -> Transport Delay/1
  Derivative/1 -> Omegadot/1

== system SimulinkOminidirectinalDrone/Vehicle Dynamic/actuator/Arm2/STANDARD ARM MODEL CLOCKWISE/PushPullDynamics ==
  Gamma reference : Inport
  Derivative : Derivative
  Derivative1 : Derivative
  G pushpull : TransferFcn  Numerator=[1212.73]  Denominator=[1 51.105 1212.73]
  Gamma : Outport
  Gammadot : Outport  Port=2
  Gammadotdot : Outport  Port=3
  wires:
  Derivative/1 -> Gammadot/1, Derivative1/1
  Derivative1/1 -> Gammadotdot/1
  Gamma reference/1 -> G pushpull/1
  G pushpull/1 -> Gamma/1, Derivative/1

== system SimulinkOminidirectinalDrone/Vehicle Dynamic/actuator/Arm2/STANDARD ARM MODEL CLOCKWISE/ServoBlockDynamics ==
  Eta reference : Inport
  Derivative : Derivative
  Derivative1 : Derivative
  G Servoblock : TransferFcn  Numerator=[1228.05]  Denominator=[1 49.1806 1228.05]
  Eta : Outport
  Etadot : Outport  Port=2
  Etadotdot : Outport  Port=3
  wires:
  Derivative/1 -> Etadot/1, Derivative1/1
  Derivative1/1 -> Etadotdot/1
  Eta reference/1 -> G Servoblock/1
  G Servoblock/1 -> Eta/1, Derivative/1

== system SimulinkOminidirectinalDrone/Vehicle Dynamic/actuator/Arm3/STANDARD ARM MODEL CLOCKWISE/Motor+ESC Dynamic ==
  Throttle reference : Inport
  Derivative : Derivative
  G Motor : TransferFcn  Numerator=[9.19]  Denominator=[0.16 1]
  Transport Delay : TransportDelay  DelayTime=0.035
  Omega : Outport
  Omegadot : Outport  Port=2
  wires:
  Transport Delay/1 -> Omega/1, Derivative/1
  Throttle reference/1 -> G Motor/1
  G Motor/1 -> Transport Delay/1
  Derivative/1 -> Omegadot/1

== system SimulinkOminidirectinalDrone/Vehicle Dynamic/actuator/Arm3/STANDARD ARM MODEL CLOCKWISE/PushPullDynamics ==
  Gamma reference : Inport
  Derivative : Derivative
  Derivative1 : Derivative
  G pushpull : TransferFcn  Numerator=[1212.73]  Denominator=[1 51.105 1212.73]
  Gamma : Outport
  Gammadot : Outport  Port=2
  Gammadotdot : Outport  Port=3
  wires:
  Derivative/1 -> Gammadot/1, Derivative1/1
  Derivative1/1 -> Gammadotdot/1
  Gamma reference/1 -> G pushpull/1
  G pushpull/1 -> Gamma/1, Derivative/1

== system SimulinkOminidirectinalDrone/Vehicle Dynamic/actuator/Arm3/STANDARD ARM MODEL CLOCKWISE/ServoBlockDynamics ==
  Eta reference : Inport
  Derivative : Derivative
  Derivative1 : Derivative
  G Servoblock : TransferFcn  Numerator=[1228.05]  Denominator=[1 49.1806 1228.05]
  Eta : Outport
  Etadot : Outport  Port=2
  Etadotdot : Outport  Port=3
  wires:
  Derivative/1 -> Etadot/1, Derivative1/1
  Derivative1/1 -> Etadotdot/1
  Eta reference/1 -> G Servoblock/1
  G Servoblock/1 -> Eta/1, Derivative/1

== system SimulinkOminidirectinalDrone/Vehicle Dynamic/actuator/Arm4/STANDARD ARM MODEL CLOCKWISE/Motor+ESC Dynamic ==
  Throttle reference : Inport
  Derivative : Derivative
  G Motor : TransferFcn  Numerator=[9.19]  Denominator=[0.16 1]
  Transport Delay : TransportDelay  DelayTime=0.035
  Omega : Outport
  Omegadot : Outport  Port=2
  wires:
  Transport Delay/1 -> Omega/1, Derivative/1
  Throttle reference/1 -> G Motor/1
  G Motor/1 -> Transport Delay/1
  Derivative/1 -> Omegadot/1

== system SimulinkOminidirectinalDrone/Vehicle Dynamic/actuator/Arm4/STANDARD ARM MODEL CLOCKWISE/PushPullDynamics ==
  Gamma reference : Inport
  Derivative : Derivative
  Derivative1 : Derivative
  G pushpull : TransferFcn  Numerator=[1212.73]  Denominator=[1 51.105 1212.73]
  Gamma : Outport
  Gammadot : Outport  Port=2
  Gammadotdot : Outport  Port=3
  wires:
  Derivative/1 -> Gammadot/1, Derivative1/1
  Derivative1/1 -> Gammadotdot/1
  Gamma reference/1 -> G pushpull/1
  G pushpull/1 -> Gamma/1, Derivative/1

== system SimulinkOminidirectinalDrone/Vehicle Dynamic/actuator/Arm4/STANDARD ARM MODEL CLOCKWISE/ServoBlockDynamics ==
  Eta reference : Inport
  Derivative : Derivative
  Derivative1 : Derivative
  G Servoblock : TransferFcn  Numerator=[1228.05]  Denominator=[1 49.1806 1228.05]
  Eta : Outport
  Etadot : Outport  Port=2
  Etadotdot : Outport  Port=3
  wires:
  Derivative/1 -> Etadot/1, Derivative1/1
  Derivative1/1 -> Etadotdot/1
  Eta reference/1 -> G Servoblock/1
  G Servoblock/1 -> Eta/1, Derivative/1

== matlab function SimulinkOminidirectinalDrone/Vehicle Dynamic/actuator/Arm4/STANDARD ARM MODEL CLOCKWISE/prop2body Matrix ==
  data: eta input; R3to1 output; gamma input
function R3to1 = prop2body(eta, gamma)
%#codegen
% Input: eta, gamma
% Output: R3to1 (3x3 rotation matrix)

R3to1 = [ cos(eta),            sin(gamma)*sin(eta),   cos(gamma)*sin(eta);
          0,                   cos(gamma),            -sin(gamma);
         -sin(eta),            cos(eta)*sin(gamma),   cos(gamma)*cos(eta) ];
end

== matlab function SimulinkOminidirectinalDrone/Vehicle Dynamic/actuator/Arm3/STANDARD ARM MODEL CLOCKWISE/MATLAB Function1 ==
  data: eta input; M output; etadot input; etadotdot input; gamma input; gammadot input; gammadotdot input; omega input; omegadot input; p input; q input; r input; pdot input; qdot input; rdot input; Ixx input; Iyy input; Izz input
function M = fcn(eta,etadot,etadotdot,gamma,gammadot,gammadotdot,omega,omegadot, p,q,r,pdot,qdot,rdot,Ixx,Iyy,Izz)

M1reactX = (1/4)*(-2*Ixx*q*r+Iyy*q*r+Izz*q*r+3*Iyy*cos(2*gamma)*q*r-3*cos(2*gamma)*q*r-...
    4*Izz*sin(gamma)*omega*r+2*Iyy*etadot*r+2*Izz*etadot+2*Iyy*cos(2*gamma)*etadot*r-2*Izz*cos(2*gamma)*etadot*r-2*Ixx*pdot-Iyy*pdot...
    -Izz*pdot+Iyy*cos(2*gamma)*pdot-Izz*cos(2*gamma)*pdot-2*Iyy*p*sin(2*gamma)*gammadot+2*Izz*p*sin(2*gamma)*gammadot...
    -sin(2*eta)*(4*(Ixx-Iyy)*p*sin(gamma)*omega+2*(Iyy-Izz)*r*sin(2*gamma)*gammadot-(2*Ixx-Iyy-Izz)*(rdot+p*(q+2*etadot))...
    -(Iyy-Izz)*cos(2*eta)*(rdot+p*(q+2*etadot)))-cos(2*eta)*(4*(Ixx-Iyy)*r*sin(gamma)*omega+2*(Izz-Iyy)*p*sin(2*gamma)*gammadot...
    +(2*Ixx-Iyy-Izz)*(pdot-r*(q+2*etadot))+(Iyy-Izz)*cos(2*gamma)*(pdot-r*(q+2*etadot)))...
    -2*cos(eta)*(2*(Ixx-Iyy+Izz)*cos(gamma)*omega*(q+etadot)+(Iyy-Izz)*sin(2*gamma)*(q-r+etadot)*...
    (q+r+etadot)+2*Ixx*gammadotdot)-2*sin(eta)*(-2*(-Ixx+Iyy+Izz)*sin(gamma)*omega*gammadot-2*Ixx*(q+etadot)*gammadot+2*(Iyy-Izz)*...
    cos(2*gamma)*(q+etadot)*gammadot+2*Izz*cos(gamma)*omegadot-(Iyy-Izz)*sin(2*gamma)*(p*r-qdot-etadotdot)));

M1reactY = (1/4)*(-2*Ixx*sin(2*eta)*p^2+Iyy*sin(2*eta)*p^2+Izz*sin(2*eta)*p^2-4*Ixx*cos(2*eta)*r*p+...
    2*Iyy*cos(2*eta)*r*p+2*Izz*cos(2*eta)*r*p-4*Ixx*sin(eta)*gammadot*p+2*Ixx*r^2*sin(2*eta)-...
    Iyy*r^2*sin*(2*eta)-Izz*r^2*sin(2*eta)-2*Iyy*qdot-2*Izz*qdot-4*Ixx*cos(eta)*r*gammadot-4*(Ixx-Iyy-Izz)*cos(gamma)*omega*(cos(eta)*p...
    -r*sin(eta)+gammadot)+2*(Iyy-Izz)*sin(2*gamma)*(-sin(eta)*(q*r+pdot)+cos(eta)*(p*q-rdot)+2*gammadot*(q+etadot))+4*Izz*sin(gamma)*...
    omegadot-2*Iyy*etadotdot-2*Izz*etadotdot-2*(Iyy-Izz)*cos(2*gamma)*(qdot+(cos(eta)*r+p*sin(eta))*(cos(eta)*p-r*sin(eta)+2*gammadot)+etadotdot));

M1reactZ = (1/4)*(-2*(Iyy-Izz)*sin(2*gamma)*sin(eta)*p^2-(4*(Iyy-Izz)*cos(2*gamma)*etadot*(sin(eta)^2+...
    (2*(-2*Ixx+Iyy+Izz)*(cos(eta)^2)-(Iyy-Izz)*cos(2*gamma)*(cos(2*eta)-3))*q...
    -4*(Izz+(Iyy-Ixx)*cos(2*eta))*sin(gamma)*omega+2*(Iyy-Izz)*cos(eta)*sin(2*gamma)*(r+2*sin(eta)*gammadot)+...
    2*(Iyy+Izz+(-2*Ixx+Iyy+Izz)*cos(2*eta))*etadot)*p-2*Ixx*rdot-Iyy*rdot-Izz*rdot+Iyy*cos(2*gamma)*...
    rdot-Izz*cos(2*gamma)*rdot-2*Iyy*r*sin(2*gamma)*gammadot+2*Izz*r*sin(2*gamma)*gammadot-cos(2*gamma)*((-2*Ixx+Iyy+Izz+(Izz-Iyy)*cos(2*gamma))*rdot+...
    2*(Iyy-Izz)*r*sin(2*gamma)*gammadot)-sin(2*eta)*(4*(Iyy-Ixx)*r*sin(gamma)*omega+(2*Ixx-Iyy-Izz)*(r*(q_2*etadot)-pdot)...
    +(Iyy-Izz)*cos(2*gamma)*(r*(q+2*etadot)-pdot))-2*sin(eta)*(-(Iyy-Izz)*sin(2*gamma)*(q+etadot)^2 ...
    -2*(Ixx-Iyy+Izz)*cos(gamma)*omega*(q+etadot)-2*Ixx*gammadotdot)-2*cos(eta)*(-2*(-Ixx+iyy+izz)*sin(gamma)*omega*gammadot...
    -2*Ixx*(q+etadot)*gammadot)+2*(Iyy-Izz)*cos(2*gamma)*(q+etadot)*gammadot+2*Izz*cos(gamma)*omegadot+(Iyy-Izz)*sin(2*gamma)*(qdot+etadotdot)));

M = [ M1reactX;
      M1reactY;
      M1reactZ];

== matlab function SimulinkOminidirectinalDrone/Vehicle Dynamic/actuator/Arm3/STANDARD ARM MODEL CLOCKWISE/prop behaviour ==
  data: Omega input; Ct input; Cq input; rho input; F output; R input; M output
function [F, M] = fcn(Omega, Ct, Cq, rho, R)
%#codegen
% Inputs:
%   rho   - air density (kg/m^3)
%   R     - propeller radius (m)
%   Omega - angular velocity (rad/s)
%   Ct    - thrust coefficient
%   Cq    - torque coefficient
%
% Outputs:
%   T - Thrust force (N)
%   Q - Torque (Nm)
% Rotor disk area
A = pi * R^2;
% Thrust (eq. 4.38)
F = rho * A * (Omega * R)^2 * Ct;
% Torque (eq. 4.39)
M = rho * A * (Omega * R)^2 * R * Cq;

end

== matlab function SimulinkOminidirectinalDrone/Vehicle Dynamic/actuator/Arm3/STANDARD ARM MODEL CLOCKWISE/prop2body Matrix ==
  data: eta input; R3to1 output; gamma input
function R3to1 = prop2body(eta, gamma)
%#codegen
% Input: eta, gamma
% Output: R3to1 (3x3 rotation matrix)

R3to1 = [ cos(eta),            sin(gamma)*sin(eta),   cos(gamma)*sin(eta);
          0,                   cos(gamma),            -sin(gamma);
         -sin(eta),            cos(eta)*sin(gamma),   cos(gamma)*cos(eta) ];
end

== matlab function SimulinkOminidirectinalDrone/Vehicle Dynamic/actuator/Arm1/STANDARD ARM MODEL CLOCKWISE/MATLAB Function1 ==
  data: eta input; M output; etadot input; etadotdot input; gamma input; gammadot input; gammadotdot input; omega input; omegadot input; p input; q input; r input; pdot input; qdot input; rdot input; Ixx input; Iyy input; Izz input
function M = fcn(eta,etadot,etadotdot,gamma,gammadot,gammadotdot,omega,omegadot, p,q,r,pdot,qdot,rdot,Ixx,Iyy,Izz)

M1reactX = (1/4)*(-2*Ixx*q*r+Iyy*q*r+Izz*q*r+3*Iyy*cos(2*gamma)*q*r-3*cos(2*gamma)*q*r-...
    4*Izz*sin(gamma)*omega*r+2*Iyy*etadot*r+2*Izz*etadot+2*Iyy*cos(2*gamma)*etadot*r-2*Izz*cos(2*gamma)*etadot*r-2*Ixx*pdot-Iyy*pdot...
    -Izz*pdot+Iyy*cos(2*gamma)*pdot-Izz*cos(2*gamma)*pdot-2*Iyy*p*sin(2*gamma)*gammadot+2*Izz*p*sin(2*gamma)*gammadot...
    -sin(2*eta)*(4*(Ixx-Iyy)*p*sin(gamma)*omega+2*(Iyy-Izz)*r*sin(2*gamma)*gammadot-(2*Ixx-Iyy-Izz)*(rdot+p*(q+2*etadot))...
    -(Iyy-Izz)*cos(2*eta)*(rdot+p*(q+2*etadot)))-cos(2*eta)*(4*(Ixx-Iyy)*r*sin(gamma)*omega+2*(Izz-Iyy)*p*sin(2*gamma)*gammadot...
    +(2*Ixx-Iyy-Izz)*(pdot-r*(q+2*etadot))+(Iyy-Izz)*cos(2*gamma)*(pdot-r*(q+2*etadot)))...
    -2*cos(eta)*(2*(Ixx-Iyy+Izz)*cos(gamma)*omega*(q+etadot)+(Iyy-Izz)*sin(2*gamma)*(q-r+etadot)*...
    (q+r+etadot)+2*Ixx*gammadotdot)-2*sin(eta)*(-2*(-Ixx+Iyy+Izz)*sin(gamma)*omega*gammadot-2*Ixx*(q+etadot)*gammadot+2*(Iyy-Izz)*...
    cos(2*gamma)*(q+etadot)*gammadot+2*Izz*cos(gamma)*omegadot-(Iyy-Izz)*sin(2*gamma)*(p*r-qdot-etadotdot)));

M1reactY = (1/4)*(-2*Ixx*sin(2*eta)*p^2+Iyy*sin(2*eta)*p^2+Izz*sin(2*eta)*p^2-4*Ixx*cos(2*eta)*r*p+...
    2*Iyy*cos(2*eta)*r*p+2*Izz*cos(2*eta)*r*p-4*Ixx*sin(eta)*gammadot*p+2*Ixx*r^2*sin(2*eta)-...
    Iyy*r^2*sin*(2*eta)-Izz*r^2*sin(2*eta)-2*Iyy*qdot-2*Izz*qdot-4*Ixx*cos(eta)*r*gammadot-4*(Ixx-Iyy-Izz)*cos(gamma)*omega*(cos(eta)*p...
    -r*sin(eta)+gammadot)+2*(Iyy-Izz)*sin(2*gamma)*(-sin(eta)*(q*r+pdot)+cos(eta)*(p*q-rdot)+2*gammadot*(q+etadot))+4*Izz*sin(gamma)*...
    omegadot-2*Iyy*etadotdot-2*Izz*etadotdot-2*(Iyy-Izz)*cos(2*gamma)*(qdot+(cos(eta)*r+p*sin(eta))*(cos(eta)*p-r*sin(eta)+2*gammadot)+etadotdot));

M1reactZ = (1/4)*(-2*(Iyy-Izz)*sin(2*gamma)*sin(eta)*p^2-(4*(Iyy-Izz)*cos(2*gamma)*etadot*(sin(eta)^2+...
    (2*(-2*Ixx+Iyy+Izz)*(cos(eta)^2)-(Iyy-Izz)*cos(2*gamma)*(cos(2*eta)-3))*q...
    -4*(Izz+(Iyy-Ixx)*cos(2*eta))*sin(gamma)*omega+2*(Iyy-Izz)*cos(eta)*sin(2*gamma)*(r+2*sin(eta)*gammadot)+...
    2*(Iyy+Izz+(-2*Ixx+Iyy+Izz)*cos(2*eta))*etadot)*p-2*Ixx*rdot-Iyy*rdot-Izz*rdot+Iyy*cos(2*gamma)*...
    rdot-Izz*cos(2*gamma)*rdot-2*Iyy*r*sin(2*gamma)*gammadot+2*Izz*r*sin(2*gamma)*gammadot-cos(2*gamma)*((-2*Ixx+Iyy+Izz+(Izz-Iyy)*cos(2*gamma))*rdot+...
    2*(Iyy-Izz)*r*sin(2*gamma)*gammadot)-sin(2*eta)*(4*(Iyy-Ixx)*r*sin(gamma)*omega+(2*Ixx-Iyy-Izz)*(r*(q_2*etadot)-pdot)...
    +(Iyy-Izz)*cos(2*gamma)*(r*(q+2*etadot)-pdot))-2*sin(eta)*(-(Iyy-Izz)*sin(2*gamma)*(q+etadot)^2 ...
    -2*(Ixx-Iyy+Izz)*cos(gamma)*omega*(q+etadot)-2*Ixx*gammadotdot)-2*cos(eta)*(-2*(-Ixx+iyy+izz)*sin(gamma)*omega*gammadot...
    -2*Ixx*(q+etadot)*gammadot)+2*(Iyy-Izz)*cos(2*gamma)*(q+etadot)*gammadot+2*Izz*cos(gamma)*omegadot+(Iyy-Izz)*sin(2*gamma)*(qdot+etadotdot)));

M = [ M1reactX;
      M1reactY;
      M1reactZ];

== matlab function SimulinkOminidirectinalDrone/Vehicle Dynamic/actuator/Arm1/STANDARD ARM MODEL CLOCKWISE/prop behaviour ==
  data: Omega input; Ct input; Cq input; rho input; F output; R input; M output
function [F, M] = fcn(Omega, Ct, Cq, rho, R)
%#codegen
% Inputs:
%   rho   - air density (kg/m^3)
%   R     - propeller radius (m)
%   Omega - angular velocity (rad/s)
%   Ct    - thrust coefficient
%   Cq    - torque coefficient
%
% Outputs:
%   T - Thrust force (N)
%   Q - Torque (Nm)
% Rotor disk area
A = pi * R^2;
% Thrust (eq. 4.38)
F = rho * A * (Omega * R)^2 * Ct;
% Torque (eq. 4.39)
M = rho * A * (Omega * R)^2 * R * Cq;

end

== matlab function SimulinkOminidirectinalDrone/Vehicle Dynamic/actuator/Arm1/STANDARD ARM MODEL CLOCKWISE/prop2body Matrix ==
  data: eta input; R3to1 output; gamma input
function R3to1 = prop2body(eta, gamma)
%#codegen
% Input: eta, gamma
% Output: R3to1 (3x3 rotation matrix)

R3to1 = [ cos(eta),            sin(gamma)*sin(eta),   cos(gamma)*sin(eta);
          0,                   cos(gamma),            -sin(gamma);
         -sin(eta),            cos(eta)*sin(gamma),   cos(gamma)*cos(eta) ];
end

== matlab function SimulinkOminidirectinalDrone/Subsystem/MATLAB Function ==
  data: B output
function B = B_matrix()
%#codegen
L     = 0.18;
H     = 0.02;
T0    = 5.0;
mu    = 1.0;
kappa = 0.01;
J     = 1.1e-4;
Omega = 450;
tr    = 0.08;
signs = [1 -1 1 -1];

B = build_B(L,H,T0,mu,kappa,J,Omega,tr,signs);

end

function B = build_B(L,H,T0,mu,kappa,J,Omega,tr,signs)
col_motor = [-L*mu; 0; kappa*L*T0; mu];
col_eta   = [-J*Omega/tr; H*T0; 0; 0];
col_gamma = [H*T0; J*Omega/tr; 0; 0];

psis = [0, pi/2, pi, 3*pi/2];
B = zeros(4,12);
for i=1:4
    psi = psis(i);
    c = cos(psi); s = sin(psi);
    Rz = [c -s 0; s c 0; 0 0 1];
    motor3 = Rz*col_motor(1:3);
    motor_col = [motor3; col_motor(4)];
    motor_col(3) = signs(i)*abs(motor_col(3));
    eta3 = Rz*col_eta(1:3);
    eta_col = [eta3;0];
    gamma3 = Rz*col_gamma(1:3);
    gamma_col = [gamma3;0];
    idx = (i-1)*3+(1:3);
    B(:,idx(1))=motor_col;
    B(:,idx(2))=eta_col;
    B(:,idx(3))=gamma_col;
end
end

== matlab function SimulinkOminidirectinalDrone/Subsystem/MATLAB Function1 ==
  data: v input; u output; B input
function u = allocator(v,B)
%#codegen
W = eye(size(B,2));        % trọng số (identity)
u = W \ B' * ((B / W * B') \ v);
end

== matlab function SimulinkOminidirectinalDrone/Vehicle Dynamic/actuator/Arm2/STANDARD ARM MODEL CLOCKWISE/prop behaviour ==
  data: Omega input; Ct input; Cq input; rho input; F output; R input; M output
function [F, M] = fcn(Omega, Ct, Cq, rho, R)
%#codegen
% Inputs:
%   rho   - air density (kg/m^3)
%   R     - propeller radius (m)
%   Omega - angular velocity (rad/s)
%   Ct    - thrust coefficient
%   Cq    - torque coefficient
%
% Outputs:
%   T - Thrust force (N)
%   Q - Torque (Nm)
% Rotor disk area
A = pi * R^2;
% Thrust (eq. 4.38)
F = rho * A * (Omega * R)^2 * Ct;
% Torque (eq. 4.39)
M = rho * A * (Omega * R)^2 * R * Cq;

end

== matlab function SimulinkOminidirectinalDrone/Vehicle Dynamic/actuator/Arm2/STANDARD ARM MODEL CLOCKWISE/prop2body Matrix ==
  data: eta input; R3to1 output; gamma input
function R3to1 = prop2body(eta, gamma)
%#codegen
% Input: eta, gamma
% Output: R3to1 (3x3 rotation matrix)

R3to1 = [ cos(eta),            sin(gamma)*sin(eta),   cos(gamma)*sin(eta);
          0,                   cos(gamma),            -sin(gamma);
         -sin(eta),            cos(eta)*sin(gamma),   cos(gamma)*cos(eta) ];
end

== matlab function SimulinkOminidirectinalDrone/Vehicle Dynamic/actuator/Arm2/STANDARD ARM MODEL CLOCKWISE/MATLAB Function1 ==
  data: eta input; M output; etadot input; etadotdot input; gamma input; gammadot input; gammadotdot input; omega input; omegadot input; p input; q input; r input; pdot input; qdot input; rdot input; Ixx input; Iyy input; Izz input
function M = fcn(eta,etadot,etadotdot,gamma,gammadot,gammadotdot,omega,omegadot, p,q,r,pdot,qdot,rdot,Ixx,Iyy,Izz)

M1reactX = (1/4)*(-2*Ixx*q*r+Iyy*q*r+Izz*q*r+3*Iyy*cos(2*gamma)*q*r-3*cos(2*gamma)*q*r-...
    4*Izz*sin(gamma)*omega*r+2*Iyy*etadot*r+2*Izz*etadot+2*Iyy*cos(2*gamma)*etadot*r-2*Izz*cos(2*gamma)*etadot*r-2*Ixx*pdot-Iyy*pdot...
    -Izz*pdot+Iyy*cos(2*gamma)*pdot-Izz*cos(2*gamma)*pdot-2*Iyy*p*sin(2*gamma)*gammadot+2*Izz*p*sin(2*gamma)*gammadot...
    -sin(2*eta)*(4*(Ixx-Iyy)*p*sin(gamma)*omega+2*(Iyy-Izz)*r*sin(2*gamma)*gammadot-(2*Ixx-Iyy-Izz)*(rdot+p*(q+2*etadot))...
    -(Iyy-Izz)*cos(2*eta)*(rdot+p*(q+2*etadot)))-cos(2*eta)*(4*(Ixx-Iyy)*r*sin(gamma)*omega+2*(Izz-Iyy)*p*sin(2*gamma)*gammadot...
    +(2*Ixx-Iyy-Izz)*(pdot-r*(q+2*etadot))+(Iyy-Izz)*cos(2*gamma)*(pdot-r*(q+2*etadot)))...
    -2*cos(eta)*(2*(Ixx-Iyy+Izz)*cos(gamma)*omega*(q+etadot)+(Iyy-Izz)*sin(2*gamma)*(q-r+etadot)*...
    (q+r+etadot)+2*Ixx*gammadotdot)-2*sin(eta)*(-2*(-Ixx+Iyy+Izz)*sin(gamma)*omega*gammadot-2*Ixx*(q+etadot)*gammadot+2*(Iyy-Izz)*...
    cos(2*gamma)*(q+etadot)*gammadot+2*Izz*cos(gamma)*omegadot-(Iyy-Izz)*sin(2*gamma)*(p*r-qdot-etadotdot)));

M1reactY = (1/4)*(-2*Ixx*sin(2*eta)*p^2+Iyy*sin(2*eta)*p^2+Izz*sin(2*eta)*p^2-4*Ixx*cos(2*eta)*r*p+...
    2*Iyy*cos(2*eta)*r*p+2*Izz*cos(2*eta)*r*p-4*Ixx*sin(eta)*gammadot*p+2*Ixx*r^2*sin(2*eta)-...
    Iyy*r^2*sin*(2*eta)-Izz*r^2*sin(2*eta)-2*Iyy*qdot-2*Izz*qdot-4*Ixx*cos(eta)*r*gammadot-4*(Ixx-Iyy-Izz)*cos(gamma)*omega*(cos(eta)*p...
    -r*sin(eta)+gammadot)+2*(Iyy-Izz)*sin(2*gamma)*(-sin(eta)*(q*r+pdot)+cos(eta)*(p*q-rdot)+2*gammadot*(q+etadot))+4*Izz*sin(gamma)*...
    omegadot-2*Iyy*etadotdot-2*Izz*etadotdot-2*(Iyy-Izz)*cos(2*gamma)*(qdot+(cos(eta)*r+p*sin(eta))*(cos(eta)*p-r*sin(eta)+2*gammadot)+etadotdot));

M1reactZ = (1/4)*(-2*(Iyy-Izz)*sin(2*gamma)*sin(eta)*p^2-(4*(Iyy-Izz)*cos(2*gamma)*etadot*(sin(eta)^2+...
    (2*(-2*Ixx+Iyy+Izz)*(cos(eta)^2)-(Iyy-Izz)*cos(2*gamma)*(cos(2*eta)-3))*q...
    -4*(Izz+(Iyy-Ixx)*cos(2*eta))*sin(gamma)*omega+2*(Iyy-Izz)*cos(eta)*sin(2*gamma)*(r+2*sin(eta)*gammadot)+...
    2*(Iyy+Izz+(-2*Ixx+Iyy+Izz)*cos(2*eta))*etadot)*p-2*Ixx*rdot-Iyy*rdot-Izz*rdot+Iyy*cos(2*gamma)*...
    rdot-Izz*cos(2*gamma)*rdot-2*Iyy*r*sin(2*gamma)*gammadot+2*Izz*r*sin(2*gamma)*gammadot-cos(2*gamma)*((-2*Ixx+Iyy+Izz+(Izz-Iyy)*cos(2*gamma))*rdot+...
    2*(Iyy-Izz)*r*sin(2*gamma)*gammadot)-sin(2*eta)*(4*(Iyy-Ixx)*r*sin(gamma)*omega+(2*Ixx-Iyy-Izz)*(r*(q_2*etadot)-pdot)...
    +(Iyy-Izz)*cos(2*gamma)*(r*(q+2*etadot)-pdot))-2*sin(eta)*(-(Iyy-Izz)*sin(2*gamma)*(q+etadot)^2 ...
    -2*(Ixx-Iyy+Izz)*cos(gamma)*omega*(q+etadot)-2*Ixx*gammadotdot)-2*cos(eta)*(-2*(-Ixx+iyy+izz)*sin(gamma)*omega*gammadot...
    -2*Ixx*(q+etadot)*gammadot)+2*(Iyy-Izz)*cos(2*gamma)*(q+etadot)*gammadot+2*Izz*cos(gamma)*omegadot+(Iyy-Izz)*sin(2*gamma)*(qdot+etadotdot)));

M = [ M1reactX;
      M1reactY;
      M1reactZ];

== matlab function SimulinkOminidirectinalDrone/Vehicle Dynamic/actuator/Arm4/STANDARD ARM MODEL CLOCKWISE/MATLAB Function1 ==
  data: eta input; M output; etadot input; etadotdot input; gamma input; gammadot input; gammadotdot input; omega input; omegadot input; p input; q input; r input; pdot input; qdot input; rdot input; Ixx input; Iyy input; Izz input
function M = fcn(eta,etadot,etadotdot,gamma,gammadot,gammadotdot,omega,omegadot, p,q,r,pdot,qdot,rdot,Ixx,Iyy,Izz)

M1reactX = (1/4)*(-2*Ixx*q*r+Iyy*q*r+Izz*q*r+3*Iyy*cos(2*gamma)*q*r-3*cos(2*gamma)*q*r-...
    4*Izz*sin(gamma)*omega*r+2*Iyy*etadot*r+2*Izz*etadot+2*Iyy*cos(2*gamma)*etadot*r-2*Izz*cos(2*gamma)*etadot*r-2*Ixx*pdot-Iyy*pdot...
    -Izz*pdot+Iyy*cos(2*gamma)*pdot-Izz*cos(2*gamma)*pdot-2*Iyy*p*sin(2*gamma)*gammadot+2*Izz*p*sin(2*gamma)*gammadot...
    -sin(2*eta)*(4*(Ixx-Iyy)*p*sin(gamma)*omega+2*(Iyy-Izz)*r*sin(2*gamma)*gammadot-(2*Ixx-Iyy-Izz)*(rdot+p*(q+2*etadot))...
    -(Iyy-Izz)*cos(2*eta)*(rdot+p*(q+2*etadot)))-cos(2*eta)*(4*(Ixx-Iyy)*r*sin(gamma)*omega+2*(Izz-Iyy)*p*sin(2*gamma)*gammadot...
    +(2*Ixx-Iyy-Izz)*(pdot-r*(q+2*etadot))+(Iyy-Izz)*cos(2*gamma)*(pdot-r*(q+2*etadot)))...
    -2*cos(eta)*(2*(Ixx-Iyy+Izz)*cos(gamma)*omega*(q+etadot)+(Iyy-Izz)*sin(2*gamma)*(q-r+etadot)*...
    (q+r+etadot)+2*Ixx*gammadotdot)-2*sin(eta)*(-2*(-Ixx+Iyy+Izz)*sin(gamma)*omega*gammadot-2*Ixx*(q+etadot)*gammadot+2*(Iyy-Izz)*...
    cos(2*gamma)*(q+etadot)*gammadot+2*Izz*cos(gamma)*omegadot-(Iyy-Izz)*sin(2*gamma)*(p*r-qdot-etadotdot)));

M1reactY = (1/4)*(-2*Ixx*sin(2*eta)*p^2+Iyy*sin(2*eta)*p^2+Izz*sin(2*eta)*p^2-4*Ixx*cos(2*eta)*r*p+...
    2*Iyy*cos(2*eta)*r*p+2*Izz*cos(2*eta)*r*p-4*Ixx*sin(eta)*gammadot*p+2*Ixx*r^2*sin(2*eta)-...
    Iyy*r^2*sin*(2*eta)-Izz*r^2*sin(2*eta)-2*Iyy*qdot-2*Izz*qdot-4*Ixx*cos(eta)*r*gammadot-4*(Ixx-Iyy-Izz)*cos(gamma)*omega*(cos(eta)*p...
    -r*sin(eta)+gammadot)+2*(Iyy-Izz)*sin(2*gamma)*(-sin(eta)*(q*r+pdot)+cos(eta)*(p*q-rdot)+2*gammadot*(q+etadot))+4*Izz*sin(gamma)*...
    omegadot-2*Iyy*etadotdot-2*Izz*etadotdot-2*(Iyy-Izz)*cos(2*gamma)*(qdot+(cos(eta)*r+p*sin(eta))*(cos(eta)*p-r*sin(eta)+2*gammadot)+etadotdot));

M1reactZ = (1/4)*(-2*(Iyy-Izz)*sin(2*gamma)*sin(eta)*p^2-(4*(Iyy-Izz)*cos(2*gamma)*etadot*(sin(eta)^2+...
    (2*(-2*Ixx+Iyy+Izz)*(cos(eta)^2)-(Iyy-Izz)*cos(2*gamma)*(cos(2*eta)-3))*q...
    -4*(Izz+(Iyy-Ixx)*cos(2*eta))*sin(gamma)*omega+2*(Iyy-Izz)*cos(eta)*sin(2*gamma)*(r+2*sin(eta)*gammadot)+...
    2*(Iyy+Izz+(-2*Ixx+Iyy+Izz)*cos(2*eta))*etadot)*p-2*Ixx*rdot-Iyy*rdot-Izz*rdot+Iyy*cos(2*gamma)*...
    rdot-Izz*cos(2*gamma)*rdot-2*Iyy*r*sin(2*gamma)*gammadot+2*Izz*r*sin(2*gamma)*gammadot-cos(2*gamma)*((-2*Ixx+Iyy+Izz+(Izz-Iyy)*cos(2*gamma))*rdot+...
    2*(Iyy-Izz)*r*sin(2*gamma)*gammadot)-sin(2*eta)*(4*(Iyy-Ixx)*r*sin(gamma)*omega+(2*Ixx-Iyy-Izz)*(r*(q_2*etadot)-pdot)...
    +(Iyy-Izz)*cos(2*gamma)*(r*(q+2*etadot)-pdot))-2*sin(eta)*(-(Iyy-Izz)*sin(2*gamma)*(q+etadot)^2 ...
    -2*(Ixx-Iyy+Izz)*cos(gamma)*omega*(q+etadot)-2*Ixx*gammadotdot)-2*cos(eta)*(-2*(-Ixx+iyy+izz)*sin(gamma)*omega*gammadot...
    -2*Ixx*(q+etadot)*gammadot)+2*(Iyy-Izz)*cos(2*gamma)*(q+etadot)*gammadot+2*Izz*cos(gamma)*omegadot+(Iyy-Izz)*sin(2*gamma)*(qdot+etadotdot)));

M = [ M1reactX;
      M1reactY;
      M1reactZ];

== matlab function SimulinkOminidirectinalDrone/Vehicle Dynamic/actuator/Arm4/STANDARD ARM MODEL CLOCKWISE/prop behaviour ==
  data: Omega input; Ct input; Cq input; rho input; F output; R input; M output
function [F, M] = fcn(Omega, Ct, Cq, rho, R)
%#codegen
% Inputs:
%   rho   - air density (kg/m^3)
%   R     - propeller radius (m)
%   Omega - angular velocity (rad/s)
%   Ct    - thrust coefficient
%   Cq    - torque coefficient
%
% Outputs:
%   T - Thrust force (N)
%   Q - Torque (Nm)
% Rotor disk area
A = pi * R^2;
% Thrust (eq. 4.38)
F = rho * A * (Omega * R)^2 * Ct;
% Torque (eq. 4.39)
M = rho * A * (Omega * R)^2 * R * Cq;

end
